simulink model "sistema_dc_dc"  (R2016a)
settings: Solver=VariableStepAuto  StartTime=0.0  StopTime=0.1  RelTol=1e-3
libraries: powerlib x13, simulink x1
settings Model: SnapshotBufferSize=20  Creator=jorda  LastModifiedBy=jorda

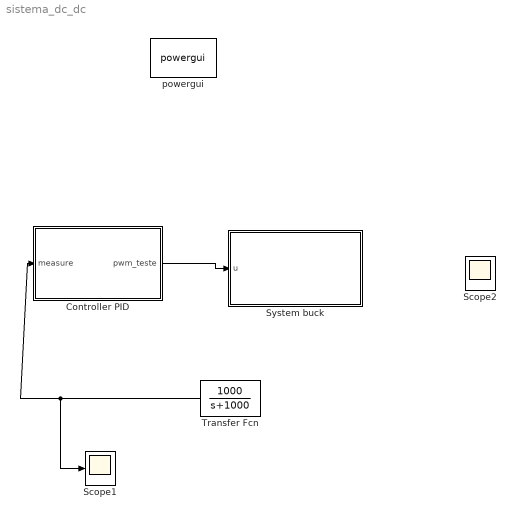
== system sistema_dc_dc ==
  Controller PID : Subsystem
  Scope1 : Scope
  Scope2 : Scope
  System buck : Subsystem
  Transfer Fcn : TransferFcn  Numerator=[1000]  Denominator=[1 1000]
  powergui : powerlib/powergui  Priority=1  SimulationMode=Continuous  SolverType=Tustin/Backward Euler (TBE)  SampleTime=50e-6  frequency=60  SPID=off  DisableSnubberDevices=off  DisableRonSwitches=off  DisableVfSwitches=off  SwTol=0  DisplayEquations=off  Interpol=off  ExternalGateDelay=off  methode=off  Ts=10  FunctionMessages=on  echomessages=on  HookPort=off  EnableUseOfTLC=off  x0status=blocks  frequencyindice=0  Pbase=100e6  ErrMax=1e-4  Iterations=50  UnitsV=V  UnitsW=MW  buscounter=0  RestoreLinks=warning  ResistiveCurrentMeasurement=off  Frange=[0:2:500]  Ylog=off  Xlog=on  ShowGrid=off  save=off  variable=ZData  structure=0  ZoomFFT=off  StartTime=0.0  cycles=1  DisplayStyle=1  fundamental=60  FreqAxis=off  MaxFrequency=1000  frequencyindicesteady=1  RmsSteady=1  display=off
  wires:
  Transfer Fcn/1 -> Scope1/1, Controller PID/1(measure)
  Controller PID/1(pwm_teste) -> System buck/1(u)
  ? -> Scope2/1, Transfer Fcn/1

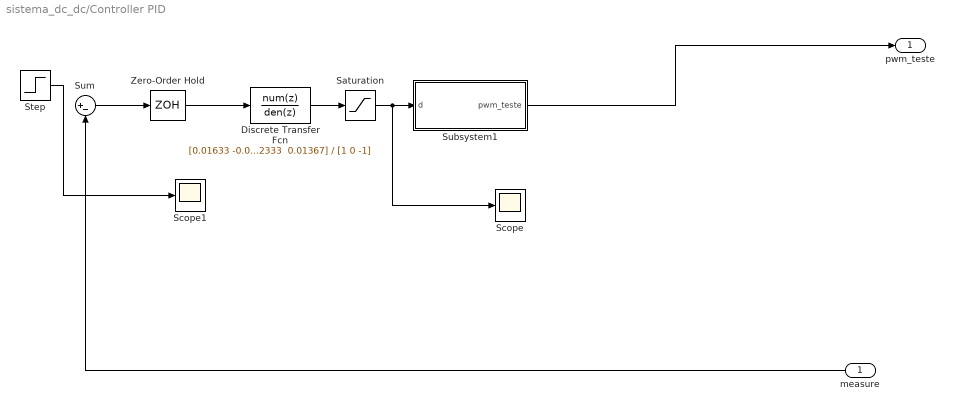
== system sistema_dc_dc/Controller PID ==
  measure : Inport
  Discrete Transfer Fcn : DiscreteTransferFcn  Numerator="[0.01633 -0.02333  0.01367]"  Denominator=[1 0 -1]  SampleTime=1e-3
  Saturation : Saturate  UpperLimit=1  LowerLimit=0
  Scope : Scope
  Scope1 : Scope
  Step : Step  Time=.5  Before=5  After=6  SampleTime=0
  Subsystem1 : Subsystem
  Sum : Sum  Inputs=|+-
  Zero-Order Hold : ZeroOrderHold  SampleTime=1e-3
  pwm_teste : Outport
  wires:
  measure/1 -> Sum/2
  Saturation/1 -> Scope/1, Subsystem1/1(d)
  Subsystem1/1(pwm_teste) -> pwm_teste/1
  Sum/1 -> Zero-Order Hold/1
  Zero-Order Hold/1 -> Discrete Transfer Fcn/1
  Discrete Transfer Fcn/1 -> Saturation/1
  Step/1 -> Scope1/1

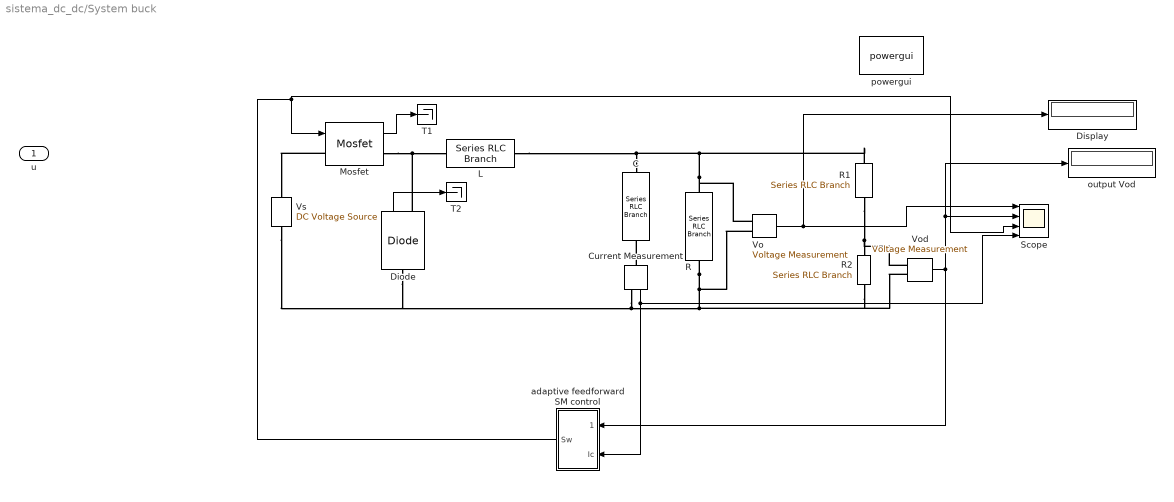
== system sistema_dc_dc/System buck ==
  u : Inport
  C : powerlib/Elements/Series RLC Branch  LConnTagsString=__new0  RConnTagsString=__new0  BranchType=C  Resistance=1  Inductance=1e-3  SetiL0=off  InitialCurrent=0  Capacitance=2000e-6  Setx0=off  InitialVoltage=0  Measurements=None
  Current Measurement : powerlib/Measurements/Current Measurement  PhasorSimulation=off  OutputType=Complex  PSBequivalent=0
  Diode : powerlib/Power Electronics/Diode  Ron=0.001  Lon=0  Vf=0.8  IC=0  UseSnubber=off  Rs=500  Cs=250e-9  Measurements=on
  Display : Display
  L : powerlib/Elements/Series RLC Branch  LConnTagsString=__new0  RConnTagsString=__new0  BranchType=L  Resistance=1  Inductance=2e-3  SetiL0=off  InitialCurrent=0  Capacitance=1e-6  Setx0=off  InitialVoltage=0  Measurements=None
  Mosfet : powerlib/Power Electronics/Mosfet  Ron=0.1  Lon=0  Rd=0.01  Vfd=0  IC=0  Rs=1e5  Cs=inf  Measurements=on
  R : powerlib/Elements/Series RLC Branch  LConnTagsString=__new0  RConnTagsString=__new0  BranchType=R  Resistance=4  Inductance=1e-3  SetiL0=off  InitialCurrent=0  Capacitance=1e-6  Setx0=off  InitialVoltage=0  Measurements=None
  R1 : powerlib/Elements/Series RLC Branch  LConnTagsString=__new0  RConnTagsString=__new0  BranchType=R  Resistance=317  Inductance=1e-3  SetiL0=off  InitialCurrent=0  Capacitance=1e-6  Setx0=off  InitialVoltage=0  Measurements=None
  R2 : powerlib/Elements/Series RLC Branch  LConnTagsString=__new0  RConnTagsString=__new0  BranchType=R  Resistance=870  Inductance=1e-3  SetiL0=off  InitialCurrent=0  Capacitance=1e-6  Setx0=off  InitialVoltage=0  Measurements=None
  Scope : Scope  NumInputPorts=4
  T1 : Terminator
  T2 : Terminator
  Vo : powerlib/Measurements/Voltage Measurement  PhasorSimulation=off  OutputType=Complex  PSBequivalent=0
  Vod : powerlib/Measurements/Voltage Measurement  PhasorSimulation=off  OutputType=Complex  PSBequivalent=0
  Vs : powerlib/Electrical Sources/DC Voltage Source  Amplitude=15  Measurements=None
  adaptive feedforward SM control : Subsystem
  output Vod : Display
  powergui : powerlib/powergui  Priority=1  SimulationMode=Continuous  SolverType=Tustin/Backward Euler (TBE)  SampleTime=50e-6  frequency=60  SPID=off  DisableSnubberDevices=off  DisableRonSwitches=off  DisableVfSwitches=off  SwTol=0  DisplayEquations=off  Interpol=off  ExternalGateDelay=off  methode=off  Ts=10  FunctionMessages=off  echomessages=off  HookPort=off  EnableUseOfTLC=off  x0status=blocks  frequencyindice=60  Pbase=100e6  ErrMax=1e-4  Iterations=50  UnitsV=kV  UnitsW=MW  buscounter=0  RestoreLinks=warning  ResistiveCurrentMeasurement=off  Frange=[0:2:500]  Ylog=off  Xlog=on  ShowGrid=off  save=off  variable=ZData  structure=0  ZoomFFT=off  StartTime=0.0  cycles=1  DisplayStyle=1  fundamental=60  FreqAxis=off  MaxFrequency=1000  frequencyindicesteady=1  RmsSteady=1  display=off
  wires:
  Diode/1 -> T2/1
  Mosfet/1 -> T1/1
  Current Measurement/1 -> Scope/4, adaptive feedforward SM control/2(Ic)
  adaptive feedforward SM control/1(Sw) -> Mosfet/1, Scope/3
  Vod/1 -> adaptive feedforward SM control/1(Vod), Scope/2, output Vod/1
  Vo/1 -> Display/1, Scope/1
  connections:
  R/LConn1 -- Vo/LConn1 -- L/RConn1 -- C/LConn1 -- R1/LConn1
  Mosfet/LConn1 -- Vs/RConn1
  R/RConn1 -- Vo/LConn2 -- R2/RConn1 -- Vod/LConn2 -- Current Measurement/RConn1 -- Vs/LConn1 -- Diode/LConn1
  Mosfet/RConn1 -- Diode/RConn1 -- L/LConn1
  R1/RConn1 -- Vod/LConn1 -- R2/LConn1
  Current Measurement/LConn1 -- C/RConn1

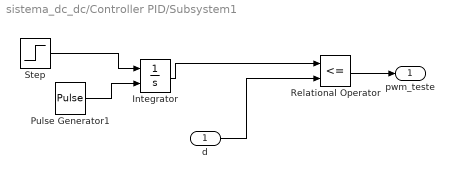
== system sistema_dc_dc/Controller PID/Subsystem1 ==
  d : Inport
  Integrator : Integrator  ExternalReset=rising
  Pulse Generator1 : DiscretePulseGenerator  PulseType=Time based  Amplitude=5  Period=1e-3  PulseWidth=50  VectorParams1D=off
  Relational Operator : RelationalOperator  Operator=<=  OutDataTypeStr=fixdt(1,16)
  Step : Step  Time=0  Before=1/1e-3  After=1/1e-3  SampleTime=0
  pwm_teste : Outport
  wires:
  Step/1 -> Integrator/1
  Pulse Generator1/1 -> Integrator/2
  Integrator/1 -> Relational Operator/1
  Relational Operator/1 -> pwm_teste/1
  d/1 -> Relational Operator/2

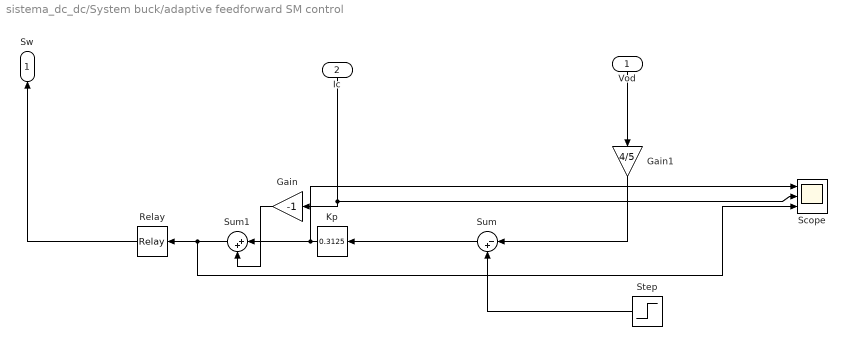
== system sistema_dc_dc/System buck/adaptive feedforward SM control ==
  Vod : Inport
  Ic : Inport  Port=2
  Gain : Gain  Gain=-1  ParamDataTypeStr=double  OutDataTypeStr=double
  Gain1 : Gain  Gain=4/5  ParamDataTypeStr=double  OutDataTypeStr=double
  Kp : simulink/Math Operations/Slider Gain  low=0  gain=0.3125  high=8000
  Relay : Relay  OnSwitchValue=0.833  OffSwitchValue=-0.833  OutDataTypeStr=Inherit: Inherit via back propagation
  Scope : Scope  NumInputPorts=3
  Step : Step  Time=0  Before=4  After=4  SampleTime=0
  Sum : Sum  Inputs=|-+  AccumDataTypeStr=single  OutDataTypeStr=double  InputSameDT=on
  Sum1 : Sum  Inputs=|++  AccumDataTypeStr=double  OutDataTypeStr=double  InputSameDT=on
  Sw : Outport
  wires:
  Gain1/1 -> Sum/1
  Ic/1 -> Scope/2, Gain/1
  Vod/1 -> Gain1/1
  Step/1 -> Sum/2
  Sum1/1 -> Scope/3, Relay/1
  Kp/1 -> Sum1/1, Scope/1
  Sum/1 -> Kp/1
  Gain/1 -> Sum1/2
  Relay/1 -> Sw/1
